simulink model "menabtrig_noio"  (Simulink 8.0)
settings: Solver=FixedStepDiscrete  StartTime=0.0  StopTime=10.0  FixedStep=1  RelTol=1e-3
settings Model: Creator=mtocci  LastModifiedBy=mtocci
settings DataIOCC: LimitDataPoints=off  SaveFormat=StructureWithTime  SignalLoggingSaveFormat=ModelDataLogs
settings OptimizationCC: InlineParams=on
settings DebuggingCC: FcnCallInpInsideContextMsg=Use local settings  StrictBusMsg=ErrorOnBusTreatedAsVector
settings GRTTargetCC: CombineOutputUpdateFcns=off

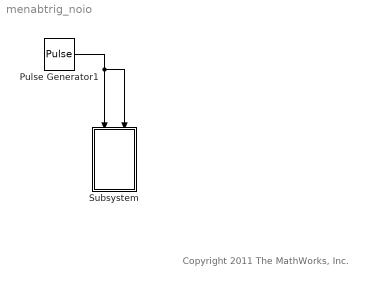
== system menabtrig_noio ==
  note: Copyright 2011 The MathWorks, Inc.
  Pulse Generator1 : DiscretePulseGenerator  Amplitude=[1 1 2 2]
  Subsystem : Subsystem
  wires:
  Pulse Generator1/1 -> Subsystem/Enable, Subsystem/Trigger

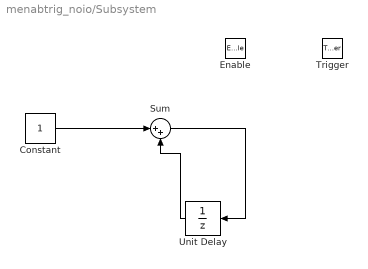
== system menabtrig_noio/Subsystem ==
  Enable : EnablePort
  Trigger : TriggerPort  PortDimensions=1
  Constant : Constant
  Sum : Sum  Inputs=|++
  Unit Delay : UnitDelay  SampleTime=-1
  wires:
  Constant/1 -> Sum/1
  Unit Delay/1 -> Sum/2
  Sum/1 -> Unit Delay/1
